simulink model "ParentTest"  (R2023a)
settings: Solver=VariableStepAuto  StartTime=0.0  StopTime=10.0  RelTol=1e-3
settings Model: Creator=Martin  LastModifiedBy=Martin

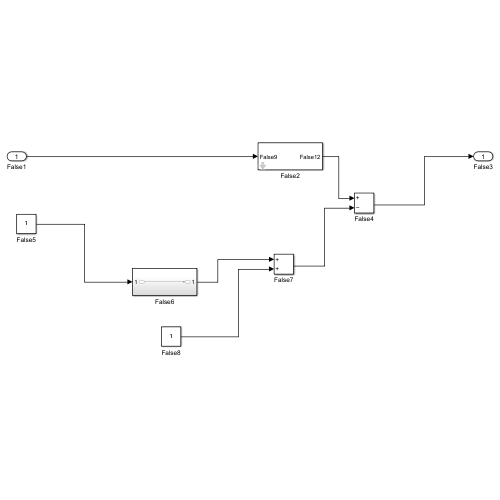
[thumbnail: Simulink's stored preview of the top-level diagram]
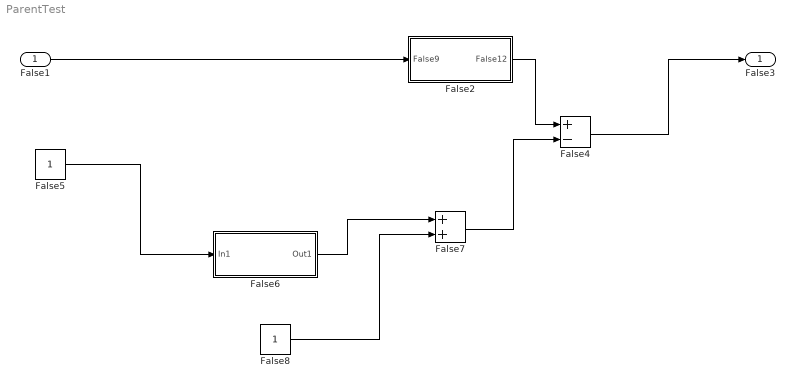
== system ParentTest ==
  False1 : Inport
  False2 : Subsystem
  False4 : Sum  Inputs=+-
  False5 : Constant
  False6 : Subsystem
  False7 : Sum
  False8 : Constant
  False3 : Outport
  wires:
  False1/1 -> False2/1(False9)
  False4/1 -> False3/1
  False6/1(Out1) -> False7/1
  False8/1 -> False7/2
  False2/1(False12) -> False4/1
  False7/1 -> False4/2
  False5/1 -> False6/1(In1)

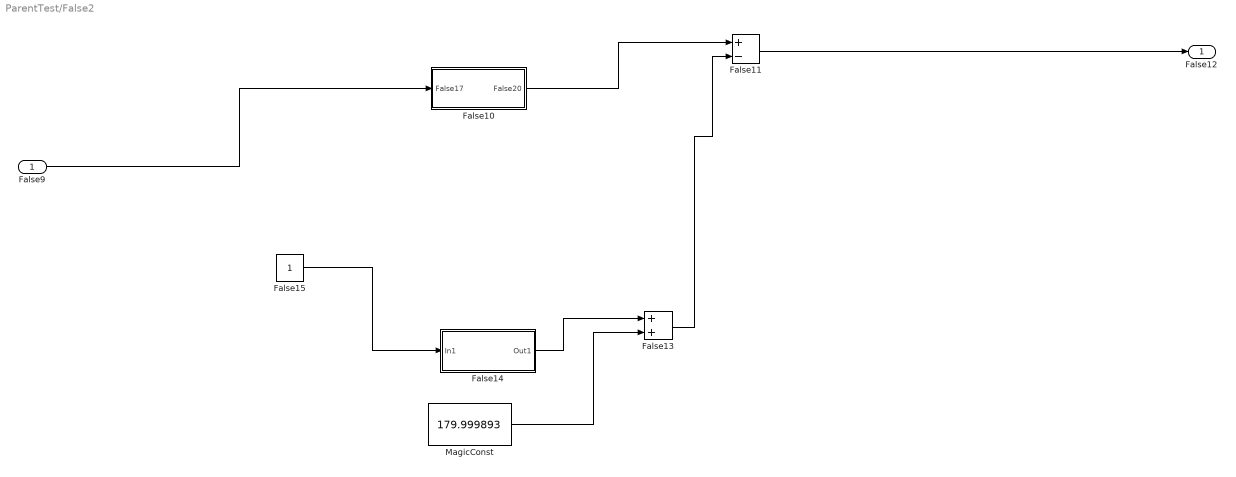
== system ParentTest/False2 ==
  False9 : Inport
  False10 : Subsystem
  False11 : Sum  Inputs=+-
  False13 : Sum
  False14 : Subsystem
  False15 : Constant
  MagicConst : Constant  Value=179.999893
  False12 : Outport
  wires:
  False15/1 -> False14/1(In1)
  False13/1 -> False11/2
  MagicConst/1 -> False13/2
  False14/1(Out1) -> False13/1
  False11/1 -> False12/1
  False10/1(False20) -> False11/1
  False9/1 -> False10/1(False17)

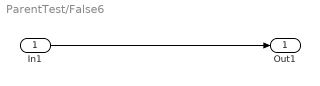
== system ParentTest/False6 ==
  In1 : Inport
  Out1 : Outport
  wires:
  In1/1 -> Out1/1

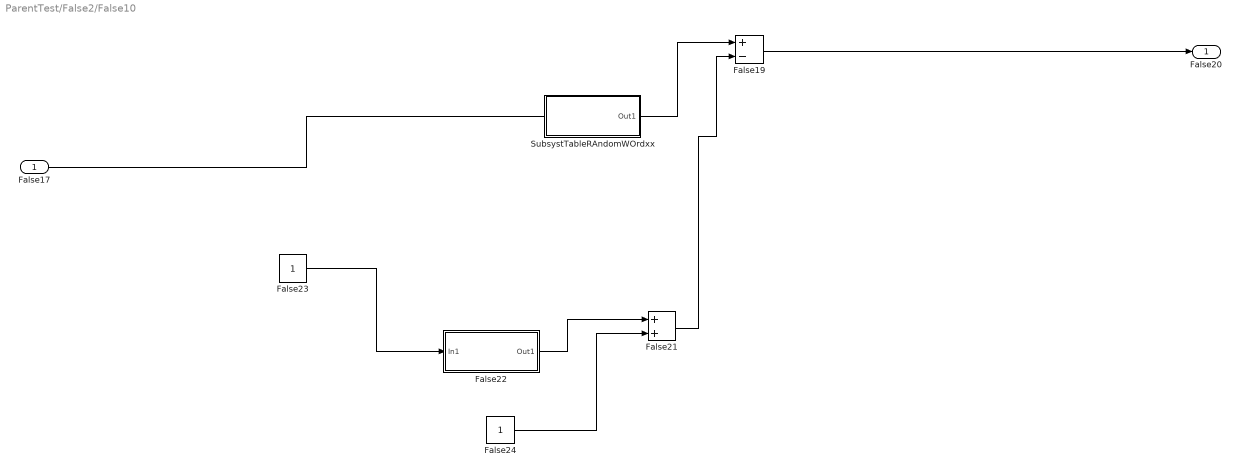
== system ParentTest/False2/False10 ==
  False17 : Inport
  False19 : Sum  Inputs=+-
  False21 : Sum
  False22 : Subsystem
  False23 : Constant
  False24 : Constant
  SubsystTableRAndomWOrdxx : Subsystem
  False20 : Outport
  wires:
  SubsystTableRAndomWOrdxx/1(Out1) -> False19/1
  False24/1 -> False21/2
  False19/1 -> False20/1
  False22/1(Out1) -> False21/1
  False21/1 -> False19/2
  False23/1 -> False22/1(In1)
  False17/1 -> ?

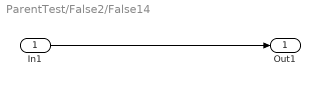
== system ParentTest/False2/False14 ==
  In1 : Inport
  Out1 : Outport
  wires:
  In1/1 -> Out1/1

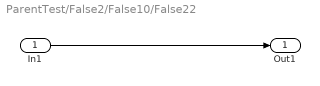
== system ParentTest/False2/False10/False22 ==
  In1 : Inport
  Out1 : Outport
  wires:
  In1/1 -> Out1/1

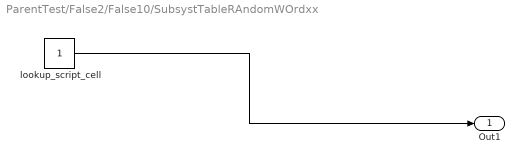
== system ParentTest/False2/False10/SubsystTableRAndomWOrdxx ==
  lookup_script_cell : Constant
  Out1 : Outport
  wires:
  lookup_script_cell/1 -> Out1/1
